simulink model "power_circ2ss_sps"  (R2023b)
settings: Solver=ode23tb  StartTime=0.0  StopTime=0.2  FixedStep=Ts  MaxStep=Ts  RelTol=1e-5
values from neighbouring files (symbols this model uses):
  sps = power_analyze('power_circ2ss_sps','structure')    [power_circ2ss_sps_calc.m]
  Ts = Ts_Control    (= 4e-05)    [HVDCMMCInterconnectionParam.m]    (also in power_circ2ss_sps_calc.m = 1e-06)
libraries: spsGroundLib x7, spsParallelRLCBranchLib x3, spsBreakerLib x2, spsVoltageMeasurementLib x2, spsControlledCurrentSourceLib x1, spsControlledVoltageSourceLib x1, spsCurrentMeasurementLib x1, spsLinearTransformerLib x1, spsMultimeterLib x1, spsSeriesRLCBranchLib x1, spspowerguiLib x1
settings Model: Creator=The MathWorks, Inc.  LastModifiedBy=rober
settings SolverCC: ZeroCrossAlgorithm=Adaptive  AlgebraicLoopSolver=TrustRegion
settings DataIOCC: SaveFormat=Array  ReturnWorkspaceOutputs=off  SignalLoggingName=sigsOut
settings OptimizationCC: BlockReduction=off  BooleanDataType=off  ExpressionDepthLimit=2147483647  InitFltsAndDblsToZero=on  EfficientMapNaN2IntZero=off  LifeSpan=inf
settings DebuggingCC: SaveWithParameterizedLinksMsg=none  UnderspecifiedInitializationDetection=Classic  MergeDetectMultiDrivingBlocksExec=none  SignalResolutionControl=TryResolveAllWithWarning  MultiTaskDSMMsg=warning  MultiTaskCondExecSysMsg=none  SigSpecEnsureSampleTimeMsg=none  FcnCallInpInsideContextMsg=warning  AllowSymbolicDim=off  StateNameClashWarn=warning  SFUnexpectedBacktrackingDiag=warning  SFNoUnconditionalDefaultTransitionDiag=warning  SFExecutionAtInitializationDiag=none  ArithmeticOperatorsInVariantConditions=warning
settings HardwareCC: ProdBitPerPointer=32  ProdBitPerSizeT=32  ProdBitPerPtrDiffT=32  ProdLargestAtomicFloat=None  ProdIntDivRoundTo=Undefined  ProdEndianess=Unspecified  ProdWordSize=32  ProdHWDeviceType=32-bit Generic  TargetUnknown=on
settings ModelReferenceCC: EnableRefExpFcnMdlSchedulingChecks=on  PropagateSignalLabelsOutOfModel=off
settings SFSimCC: SimUseLocalCustomCode=off  CustomCodeUndefinedFunction=UseInterfaceOnly
settings RTWCC: RTWUseLocalCustomCode=off  DLArmComputeVersion=19.05
settings CodeAppCC: StateflowObjectComments=on
settings GRTTargetCC: TargetFcnLib=ansi_tfl_tmw.mat  TargetLangStandard=C89/C90 (ANSI)  CombineOutputUpdateFcns=off  GRTInterface=on
settings ConfigComp: CovMetricSettings=dw  CovSaveCumulativeToWorkspaceVar=on  CovSaveSingleToWorkspaceVar=on  CovExternalEMLEnable=off  CovSFcnEnable=off
settings SimscapeCC: SimscapeNormalizeSystem=off

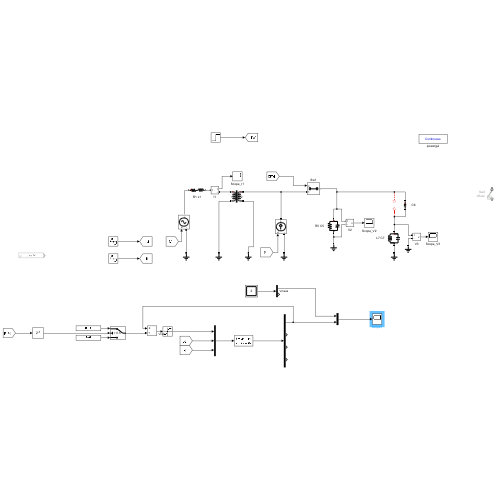
[thumbnail: Simulink's stored preview of the top-level diagram]
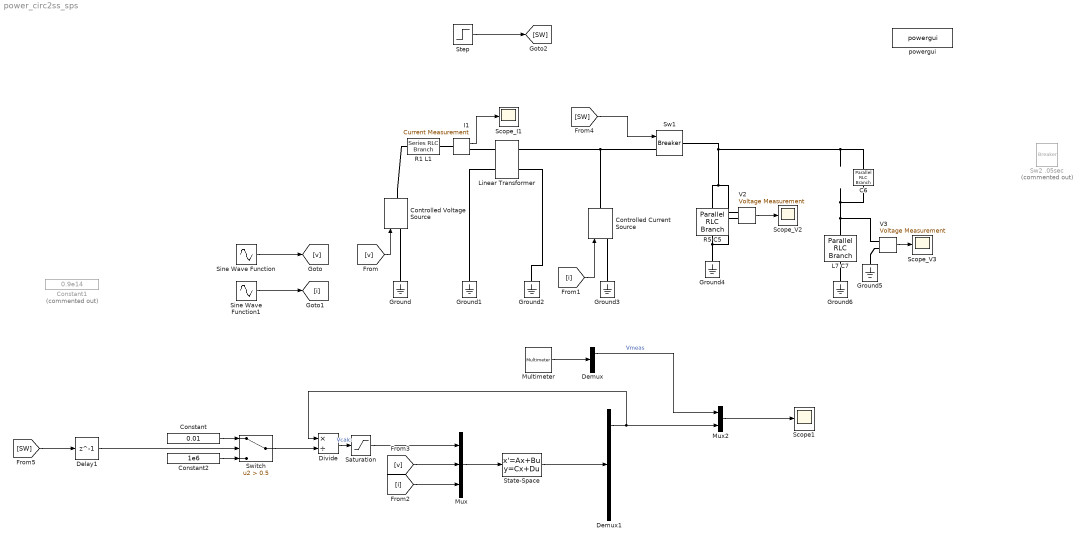
== system power_circ2ss_sps ==
  C6 : spsParallelRLCBranchLib/Parallel RLC Branch  LConnTagsString=a  RConnTagsString=__new0  BranchType=C  Resistance=[]  Inductance=[]  SetiL0=off  InitialCurrent=0  Capacitance=1e-09  Setx0=off  InitialVoltage=0  Measurements=None
  Constant : Constant  Value=0.01
  Constant1 : Constant  Commented=on  Value=0.9e14
  Constant2 : Constant  Value=1e6
  Controlled Current Source : spsControlledCurrentSourceLib/Controlled Current Source  Initialize=on  Source_Type=AC  Amplitude=0  Phase=0  Frequency=0  Measurements=None
  Controlled Voltage Source : spsControlledVoltageSourceLib/Controlled Voltage Source  Initialize=on  Source_Type=AC  Amplitude=0  Phase=0  Frequency=0  Measurements=None
  Delay1 : Delay  DelayLength=1
  Demux : Demux  Outputs=2
  Demux1 : Demux  Outputs=numel(sps.outputs)
  Divide : Product  Inputs=*/
  Ground{,1..6} (7 alike) : spsGroundLib/Ground  LConnTagsString=a
  I1 : spsCurrentMeasurementLib/Current Measurement  Tag=PoWeRsYsTeMmEaSuReMeNt  PhasorSimulation=off  OutputType=Magnitude  PSBequivalent=0
      settings: AttributesFormatString=\n
  L7 C7 : spsParallelRLCBranchLib/Parallel RLC Branch  LConnTagsString=a  RConnTagsString=__new0  BranchType=LC  Resistance=[]  Inductance=0.5  SetiL0=off  InitialCurrent=0  Capacitance=2e-06  Setx0=off  InitialVoltage=0  Measurements=None
  Linear Transformer : spsLinearTransformerLib/Linear Transformer  UNITS=pu  NominalPower=[10000 60]  winding1=[100 0.05 1.5e-3*377]  winding2=[200 0.05 0]  ThreeWindings=off  winding3=[3.15e+05 0.002 0.08]  RmLm=[499.98 500]  Measurements=None  DataType=off
  Multimeter : spsMultimeterLib/Multimeter  L=2  sel=[1 2]  yselected={}  Gain=[1 1]  OutputType=Complex  PlotAtSimulationStop=off  PhasorSimulation=off
  Mux : Mux  Inputs=numel(sps.inputs)
  Mux2 : Mux  Inputs=2
  R1 L1 : spsSeriesRLCBranchLib/Series RLC Branch  LConnTagsString=__new0  RConnTagsString=__new0  BranchType=RL  Resistance=0.1  Inductance=1e-03  SetiL0=off  InitialCurrent=0  Capacitance=[]  Setx0=off  InitialVoltage=0  Measurements=None
  R5 C5 : spsParallelRLCBranchLib/Parallel RLC Branch  LConnTagsString=a  RConnTagsString=__new0  BranchType=RC  Resistance=200  Inductance=[]  SetiL0=off  InitialCurrent=0  Capacitance=1e-06  Setx0=off  InitialVoltage=0  Measurements=None
  Saturation : Saturate  UpperLimit=2  LowerLimit=-2
  Scope1 : Scope
  Scope_I1 : Scope
  Scope_V2 : Scope
  Scope_V3 : Scope
  Sine Wave Function : Sin  Amplitude=100  Frequency=2*pi*60  SampleTime=Ts
  Sine Wave Function1 : Sin  Amplitude=2  Frequency=2*pi*180  Phase=deg2rad(30)  SampleTime=Ts
  State-Space : StateSpace  A=sps.A  B=sps.B  C=sps.C  D=sps.D  InitialCondition=sps.x0
  Step : Step  Time=0.1  SampleTime=0
  Sw1 : spsBreakerLib/Breaker  InitialState=1  SwitchingTimes="[ .1  ]"  External=on  BreakerResistance=0.01  SnubberResistance=1e6  SnubberCapacitance=0  Measurements=Branch voltage and current  MoreParameters=off  NoBreakLoop=off
      settings: AttributesFormatString=\n
  Sw2 .05sec : spsBreakerLib/Breaker  Commented=on  InitialState=0  SwitchingTimes=[ .05 ]  External=off  BreakerResistance=0.1  SnubberResistance=inf  SnubberCapacitance=0  Measurements=None  MoreParameters=off  NoBreakLoop=off
      settings: AttributesFormatString=\n
  Switch : Switch  Criteria=u2 > Threshold  Threshold=0.5  SaturateOnIntegerOverflow=off  InputSameDT=off
  V2 : spsVoltageMeasurementLib/Voltage Measurement  Tag=PoWeRsYsTeMmEaSuReMeNt  PhasorSimulation=off  OutputType=Magnitude  PSBequivalent=0
  V3 : spsVoltageMeasurementLib/Voltage Measurement  Tag=PoWeRsYsTeMmEaSuReMeNt  PhasorSimulation=off  OutputType=Magnitude  PSBequivalent=0
  powergui : spspowerguiLib/powergui  Priority=2  SimulationMode=Continuous  SampleTime=Ts  frequency=60  Iterations=50  frequencyindice=0  Pbase=100e6  ErrMax=1e-4  UnitsV=kV  UnitsW=MW  buscounter=0  FunctionMessages=off  echomessages=off  EnableUseOfTLC=off  CurrentSourceSwitches=on  DisableSnubberDevices=off  DisableRonSwitches=off  DisableVfSwitches=off  DisplayEquations=off  AutomaticDiscreteSolvers=off  SolverType=Tustin/Backward Euler (TBE)  Interpol=off  ExternalGateDelay=off  methode=off  Ts=0  x0status=blocks  SPID=off  SwTol=0  HookPort=off  NonlinearTolerance=1e-4  nMaxIteration=100  ContinueOnMaxIteration=off  RestoreLinks=warning  ResistiveCurrentMeasurement=off  Frange=logspace(0,3,50)  Ylog=off  Xlog=off  ShowGrid=off  save=off  variable=ZData  structure=0  ZoomFFT=on  StartTime=0.0  cycles=1  DisplayStyle=off  fundamental=60  FreqAxis=off  MaxFrequency=1000  frequencyindicesteady=1  RmsSteady=1  display=off
  wires:
  I1/1 -> Scope_I1/1
  V3/1 -> Scope_V3/1
  V2/1 -> Scope_V2/1
  Sine Wave Function/1 -> [v]
  [i] -> Controlled Current Source/1
  Mux/1 -> State-Space/1
  [v] -> Controlled Voltage Source/1
  Sine Wave Function1/1 -> [i]
  [i] -> Mux/3
  [v] -> Mux/2
  Multimeter/1 -> Demux/1
  [SW] -> Sw1/1
  Step/1 -> [SW]
  [SW] -> Delay1/1
  Constant2/1 -> Switch/3
  Constant/1 -> Switch/1
  Switch/1 -> Divide/2
  Divide/1 -> Saturation/1  "Vcalc"
  Mux2/1 -> Scope1/1
  Demux1/1 -> Mux2/2, Divide/1
  State-Space/1 -> Demux1/1
  Saturation/1 -> Mux/1
  Delay1/1 -> Switch/2
  Demux/1 -> Mux2/1  "Vmeas"
  connections:
  Controlled Voltage Source/RConn1 -- R1 L1/LConn1
  Ground/LConn1 -- Controlled Voltage Source/LConn1
  Linear Transformer/RConn2 -- Ground2/LConn1
  Linear Transformer/LConn2 -- Ground1/LConn1
  Sw1/LConn1 -- Controlled Current Source/RConn1 -- Linear Transformer/RConn1
  R1 L1/RConn1 -- I1/LConn1
  Linear Transformer/LConn1 -- I1/RConn1
  C6/RConn1 -- L7 C7/LConn1 -- V3/LConn1
  Ground5/LConn1 -- V3/LConn2
  Ground4/LConn1 -- R5 C5/RConn1 -- V2/LConn2
  Sw1/RConn1 -- R5 C5/LConn1 -- V2/LConn1 -- C6/LConn1
  Ground3/LConn1 -- Controlled Current Source/LConn1
  L7 C7/RConn1 -- Ground6/LConn1
